simulink model "Simulation_Fahrmodell_v3"  (R2023b)
settings: Solver=ode14x  StartTime=0.0  StopTime=600  FixedStep=0.005  RelTol=1e-3
values from neighbouring files (symbols this model uses):
  bat = bat.computePack()    [DoE_main.m]    (also in DoE_main_sensitivity.m)
  cp = cp.computeP4Map(val_P4, 0, val_P4_DM, 0, 0)    [DoE_main.m]    (also in DoE_main_sensitivity.m = cp.computeP4Map(P4, E2, P4_DM, E3, E4))
  gb = gb.computeShiftMaps()    [DoE_main.m]    (also in DoE_main_sensitivity.m)
  P4 = cfgNum(cfg, 'P4', 0)    [DoE_main_sensitivity.m]    (also in PowertrainConfig.m = 0)
  P4_DM = cfgNum(cfg, 'P4_DM', 0)    [DoE_main_sensitivity.m]    (also in PowertrainConfig.m = 0)
  pt = pt.setupHybrid()    [DoE_main.m]    (also in DoE_main_sensitivity.m)
  veh = VehicleConfig()    [DoE_main.m]    (also in DoE_main_sensitivity.m)
undefined symbols (not defined in the file or in its folder): cp_Zelle_JpkgK, Ice_derfacLoadDecrease_MAP, Ice_derfacLoadIncrease_MAP, Ice_n_axis, Ice_relLoadMax_CUR_n, Ice_relLoadMax_CUR_val, Ice_rl_axis_norm, seconds, SKO_STREET_CHAL, SKO_WHEEL_TYP_CHAL, slip_pacejka, T_init_degC, Track, TT_sliced, use_turbo_model, v_Fzg_init_kmph
libraries: nesl_utility x15, fl_lib x9
(part 5 of 6)

== system Simulation_Fahrmodell_v3/Vehicle Dynamics Model /Drivetrain/Primary and Secondary Axle Powertrain Selector/Primary Axle Powertrain Selector/Hybrid Drive/P2/P2 Motor/Battery and Operating Strategy Limitation (Drive) ==
  Motordrehzahl (1/min) : Inport
  tq_sh_P2_limted : Inport  Port=2
  P_max_EM_kW : Inport  Port=3
  "Begrenzung BAT + Betriebsstrategie EM P2, Fahren1" : Subsystem
  Discharge Limit : Subsystem
  n_Upmin OUT : Outport
  tq_sh_P2_bat_limted : Outport  Port=2
  wires:
  "Begrenzung BAT + Betriebsstrategie EM P2, Fahren1"/2(M_begr_Nm) -> tq_sh_P2_bat_limted/1  "P2_M_Nm_Fahren"
  tq_sh_P2_limted/1 -> Discharge Limit/1(Torque_Drive_In)
  Motordrehzahl (1/min)/1 -> "Begrenzung BAT + Betriebsstrategie EM P2, Fahren1"/1(n_Upmin IN)
  Discharge Limit/1(Torque_Drive_Out) -> "Begrenzung BAT + Betriebsstrategie EM P2, Fahren1"/2(M_Nm)  "P2_M_Nm_Fahren"
  P_max_EM_kW/1 -> "Begrenzung BAT + Betriebsstrategie EM P2, Fahren1"/3(P_mech_max_kW)
  "Begrenzung BAT + Betriebsstrategie EM P2, Fahren1"/1(n_Upmin OUT) -> n_Upmin OUT/1

== system Simulation_Fahrmodell_v3/Vehicle Dynamics Model /Drivetrain/Primary and Secondary Axle Powertrain Selector/Primary Axle Powertrain Selector/Hybrid Drive/P2/P2 Motor/Battery and Operating Strategy Limitation (Recuperation) ==
  Motordrehzahl (1/min) : Inport
  Torque_Recu_In : Inport  Port=2
  P_min_EM_kW : Inport  Port=3
  "Begrenzung BAT + Betriebsstrategie EM P2, Reku1" : Subsystem
  Recuperation Limit1 : Subsystem
  n_Upmin OUT : Outport
  tq_sh_P2_bat_limted_recu : Outport  Port=2
  wires:
  Recuperation Limit1/1(Torque_Recu_Out) -> "Begrenzung BAT + Betriebsstrategie EM P2, Reku1"/2(M_Nm)  "P2_M_Nm_Reku"
  Torque_Recu_In/1 -> Recuperation Limit1/1(Torque_Recu_In)
  "Begrenzung BAT + Betriebsstrategie EM P2, Reku1"/2(M_begr_Nm) -> tq_sh_P2_bat_limted_recu/1  "P2_M_Nm_Reku"
  P_min_EM_kW/1 -> "Begrenzung BAT + Betriebsstrategie EM P2, Reku1"/3(P_mech_max_kW)
  Motordrehzahl (1/min)/1 -> "Begrenzung BAT + Betriebsstrategie EM P2, Reku1"/1(n_Upmin IN)
  "Begrenzung BAT + Betriebsstrategie EM P2, Reku1"/1(n_Upmin OUT) -> n_Upmin OUT/1

== system Simulation_Fahrmodell_v3/Vehicle Dynamics Model /Drivetrain/Primary and Secondary Axle Powertrain Selector/Primary Axle Powertrain Selector/Hybrid Drive/P2/P2 Motor/Power Calculation ==
  n_Upmin : Inport
  tq_sh_P2_bat_limted : Inport  Port=2
  Constant1 : Constant  Value=2*pi/60/1000
  Product : Product  Inputs=3
  P_kW : Outport
  wires:
  Product/1 -> P_kW/1
  n_Upmin/1 -> Product/2
  Constant1/1 -> Product/3
  tq_sh_P2_bat_limted/1 -> Product/1

== system Simulation_Fahrmodell_v3/Vehicle Dynamics Model /Drivetrain/Primary and Secondary Axle Powertrain Selector/Primary Axle Powertrain Selector/Hybrid Drive/P2/P2 Motor/Power Calculation  ==
  n_Upmin : Inport
  tq_sh_P2_bat_limted_recu : Inport  Port=2
  Constant1 : Constant  Value=2*pi/60/1000
  Product : Product  Inputs=3
  P_kW : Outport
  wires:
  Product/1 -> P_kW/1
  n_Upmin/1 -> Product/2
  Constant1/1 -> Product/3
  tq_sh_P2_bat_limted_recu/1 -> Product/1

== system Simulation_Fahrmodell_v3/Vehicle Dynamics Model /Drivetrain/Primary and Secondary Axle Powertrain Selector/Primary Axle Powertrain Selector/Hybrid Drive/P3/P3 Motor/Battery and Operating Strategy Limitation (Drive) ==
  n_Upmin IN : Inport
  tq_sh_P3_limted : Inport  Port=2
  P_max_EM_kW : Inport  Port=3
  "Begrenzung BAT + Betriebsstrategie EM P2, Fahren1" : Subsystem
  Discharge Limit : Subsystem
  n_Upmin OUT : Outport
  tq_sh_P3_bat_limted : Outport  Port=2
  wires:
  P_max_EM_kW/1 -> "Begrenzung BAT + Betriebsstrategie EM P2, Fahren1"/3(P_max_EM_kW)
  tq_sh_P3_limted/1 -> Discharge Limit/1(Torque_Drive_In)
  Discharge Limit/1(Torque_Drive_Out) -> "Begrenzung BAT + Betriebsstrategie EM P2, Fahren1"/2(M_Nm)  "P4_M_Nm_Fahren"
  n_Upmin IN/1 -> "Begrenzung BAT + Betriebsstrategie EM P2, Fahren1"/1(n_Upmin IN)
  "Begrenzung BAT + Betriebsstrategie EM P2, Fahren1"/2(tq_sh_P3_bat_limted) -> tq_sh_P3_bat_limted/1
  "Begrenzung BAT + Betriebsstrategie EM P2, Fahren1"/1(n_Upmin OUT) -> n_Upmin OUT/1

== system Simulation_Fahrmodell_v3/Vehicle Dynamics Model /Drivetrain/Primary and Secondary Axle Powertrain Selector/Primary Axle Powertrain Selector/Hybrid Drive/P3/P3 Motor/Battery and Operating Strategy Limitation (Recuperation) ==
  n_Upmin IN : Inport
  Torque_Recu_In : Inport  Port=2
  P_mech_max_kW : Inport  Port=3
  "Begrenzung BAT + Betriebsstrategie EM P2, Reku1" : Subsystem
  Recuperation Limit1 : Subsystem
  n_Upmin OUT : Outport
  tq_sh_P3_bat_limted : Outport  Port=2
  wires:
  Recuperation Limit1/1(Torque_Recu_Out) -> "Begrenzung BAT + Betriebsstrategie EM P2, Reku1"/2(M_Nm)  "P3_M_Nm_Reu"
  Torque_Recu_In/1 -> Recuperation Limit1/1(Torque_Recu_In)
  n_Upmin IN/1 -> "Begrenzung BAT + Betriebsstrategie EM P2, Reku1"/1(n_Upmin IN)
  "Begrenzung BAT + Betriebsstrategie EM P2, Reku1"/2(M_begr_Nm) -> tq_sh_P3_bat_limted/1
  P_mech_max_kW/1 -> "Begrenzung BAT + Betriebsstrategie EM P2, Reku1"/3(P_mech_max_kW)
  "Begrenzung BAT + Betriebsstrategie EM P2, Reku1"/1(n_Upmin OUT) -> n_Upmin OUT/1

== system Simulation_Fahrmodell_v3/Vehicle Dynamics Model /Drivetrain/Primary and Secondary Axle Powertrain Selector/Primary Axle Powertrain Selector/Hybrid Drive/P3/P3 Motor/Power Calculation ==
  n_Upmin : Inport
  tq_sh_P3_bat_limted : Inport  Port=2
  Constant1 : Constant  Value=2*pi/60/1000
  Product : Product  Inputs=3
  P_max_EM_P3_kW : Outport
  wires:
  Product/1 -> P_max_EM_P3_kW/1
  n_Upmin/1 -> Product/2
  Constant1/1 -> Product/3
  tq_sh_P3_bat_limted/1 -> Product/1

== system Simulation_Fahrmodell_v3/Vehicle Dynamics Model /Drivetrain/Primary and Secondary Axle Powertrain Selector/Primary Axle Powertrain Selector/Hybrid Drive/P3/P3 Motor/Power Calculation  ==
  n_Upmin : Inport
  tq_sh_P3_bat_limted : Inport  Port=2
  Constant1 : Constant  Value=2*pi/60/1000
  Product : Product  Inputs=3
  P_kW : Outport
  wires:
  Product/1 -> P_kW/1
  n_Upmin/1 -> Product/2
  Constant1/1 -> Product/3
  tq_sh_P3_bat_limted/1 -> Product/1

== system Simulation_Fahrmodell_v3/Vehicle Dynamics Model /Drivetrain/Primary and Secondary Axle Powertrain Selector/Secondary Axle Powertrain Selector/Auswahl P4, P4_Dual-Motor/P4 // E2 Single Motor/Battery and Operating Strategy Limitation (Drive)/Begrenzung BAT + Betriebsstrategie EM P4, Fahren1 ==
  n_Upmin IN : Inport
  M_Nm : Inport  Port=2
  P_mech_max_kW : Inport  Port=3
  Max1 : MinMax  Inputs=2
  "P_kW -> M_Nm" : Subsystem
  n_Upmin OUT : Outport
  M_begr_Nm : Outport  Port=2
  wires:
  M_Nm/1 -> Max1/1
  Max1/1 -> M_begr_Nm/1
  "P_kW -> M_Nm"/1(Out1) -> Max1/2  "M_mech_max_Nm"
  n_Upmin IN/1 -> "P_kW -> M_Nm"/2(In2), n_Upmin OUT/1
  P_mech_max_kW/1 -> "P_kW -> M_Nm"/1(P_kW)  "P_kW"

== system Simulation_Fahrmodell_v3/Vehicle Dynamics Model /Drivetrain/Primary and Secondary Axle Powertrain Selector/Secondary Axle Powertrain Selector/Auswahl P4, P4_Dual-Motor/P4 // E2 Single Motor/Battery and Operating Strategy Limitation (Drive)/Discharge Limit ==
  Torque_Drive_In : Inport
  Gain2 : Gain  Gain=100
  MATLAB Function : MATLAB Function  TreatAsAtomicUnit=on
  Recuperation Limit2 : Constant  Value=bat.SOC_Bat_Discharge_Limit
  Torque_Drive_Out : Outport
  wires:
  Torque_Drive_In/1 -> MATLAB Function/1(Torque_In)
  Recuperation Limit2/1 -> Gain2/1
  MATLAB Function/1(Torque_Out) -> Torque_Drive_Out/1
  [SOC] -> MATLAB Function/2(SOC)
  Gain2/1 -> MATLAB Function/3(Discharge_Limit)

== system Simulation_Fahrmodell_v3/Vehicle Dynamics Model /Drivetrain/Primary and Secondary Axle Powertrain Selector/Secondary Axle Powertrain Selector/Auswahl P4, P4_Dual-Motor/P4 // E2 Single Motor/Battery and Operating Strategy Limitation (Recuperation)/Begrenzung BAT + Betriebsstrategie EM P4, Reku1 ==
  n_Upmin IN : Inport
  M_Nm : Inport  Port=2
  P_mech_max_kW : Inport  Port=3
  Max1 : MinMax  Function=max  Inputs=2
  "P_kW -> M_Nm" : Subsystem
  n_Upmin OUT : Outport
  M_begr_Nm : Outport  Port=2
  wires:
  M_Nm/1 -> Max1/1
  Max1/1 -> M_begr_Nm/1
  "P_kW -> M_Nm"/1(Out1) -> Max1/2  "M_mech_max_Nm"
  n_Upmin IN/1 -> "P_kW -> M_Nm"/2(In2), n_Upmin OUT/1
  P_mech_max_kW/1 -> "P_kW -> M_Nm"/1(P_kW)  "P_kW"

== system Simulation_Fahrmodell_v3/Vehicle Dynamics Model /Drivetrain/Primary and Secondary Axle Powertrain Selector/Secondary Axle Powertrain Selector/Auswahl P4, P4_Dual-Motor/P4 // E2 Single Motor/Battery and Operating Strategy Limitation (Recuperation)/Recuperation Limit ==
  Torque_Recu_In : Inport
  Constant : Constant  Value=0
  Gain5 : Gain  Gain=100
  Recuperation Limit : Constant  Value=bat.SOC_Recup_Limit
  Relational Operator2 : RelationalOperator  Operator=<  OutDataTypeStr=boolean  RndMeth=Simplest  InputSameDT=off
  Switch2 : Switch  Criteria=u2 > Threshold  SaturateOnIntegerOverflow=off  InputSameDT=off
  Torque_Recu_Out : Outport
  wires:
  Constant/1 -> Switch2/3
  [SOC] -> Relational Operator2/1
  Recuperation Limit/1 -> Gain5/1
  Relational Operator2/1 -> Switch2/2
  Torque_Recu_In/1 -> Switch2/1
  Switch2/1 -> Torque_Recu_Out/1
  Gain5/1 -> Relational Operator2/2

== system Simulation_Fahrmodell_v3/Vehicle Dynamics Model /Drivetrain/Primary and Secondary Axle Powertrain Selector/Secondary Axle Powertrain Selector/Auswahl P4, P4_Dual-Motor/P4 // E3 // E4 Dual Motor/Battery and Operating Strategy Limitation (Drive) 1/Begrenzung BAT + Betriebsstrategie EM P4_DM_L, Fahren1 ==
  n_Upmin IN : Inport
  M_Nm : Inport  Port=2
  P_mech_max_kW : Inport  Port=3
  Max1 : MinMax  Inputs=2
  "P_kW -> M_Nm" : Subsystem
  n_Upmin OUT : Outport
  M_begr_Nm : Outport  Port=2
  wires:
  M_Nm/1 -> Max1/1
  Max1/1 -> M_begr_Nm/1
  "P_kW -> M_Nm"/1(Out1) -> Max1/2  "M_mech_max_Nm"
  n_Upmin IN/1 -> "P_kW -> M_Nm"/2(In2), n_Upmin OUT/1
  P_mech_max_kW/1 -> "P_kW -> M_Nm"/1(P_kW)  "P_kW"

== system Simulation_Fahrmodell_v3/Vehicle Dynamics Model /Drivetrain/Primary and Secondary Axle Powertrain Selector/Secondary Axle Powertrain Selector/Auswahl P4, P4_Dual-Motor/P4 // E3 // E4 Dual Motor/Battery and Operating Strategy Limitation (Drive) 1/Discharge Limit1 ==
  Torque_Drive_In : Inport
  Gain2 : Gain  Gain=100
  MATLAB Function : MATLAB Function  TreatAsAtomicUnit=on
  Recuperation Limit2 : Constant  Value=bat.SOC_Bat_Discharge_Limit
  Torque_Drive_Out : Outport
  wires:
  Torque_Drive_In/1 -> MATLAB Function/1(Torque_In)
  Recuperation Limit2/1 -> Gain2/1
  MATLAB Function/1(Torque_Out) -> Torque_Drive_Out/1
  [SOC] -> MATLAB Function/2(SOC)
  Gain2/1 -> MATLAB Function/3(Discharge_Limit)

== system Simulation_Fahrmodell_v3/Vehicle Dynamics Model /Drivetrain/Primary and Secondary Axle Powertrain Selector/Secondary Axle Powertrain Selector/Auswahl P4, P4_Dual-Motor/P4 // E3 // E4 Dual Motor/Battery and Operating Strategy Limitation (Drive) 2/Begrenzung BAT + Betriebsstrategie EM P4_DM_R, Fahren2 ==
  n_Upmin IN : Inport
  M_Nm : Inport  Port=2
  P_mech_max_kW : Inport  Port=3
  Max1 : MinMax  Inputs=2
  "P_kW -> M_Nm" : Subsystem
  n_Upmin OUT : Outport
  M_begr_Nm : Outport  Port=2
  wires:
  M_Nm/1 -> Max1/1
  Max1/1 -> M_begr_Nm/1
  "P_kW -> M_Nm"/1(Out1) -> Max1/2  "M_mech_max_Nm"
  n_Upmin IN/1 -> "P_kW -> M_Nm"/2(In2), n_Upmin OUT/1
  P_mech_max_kW/1 -> "P_kW -> M_Nm"/1(P_kW)  "P_kW"

== system Simulation_Fahrmodell_v3/Vehicle Dynamics Model /Drivetrain/Primary and Secondary Axle Powertrain Selector/Secondary Axle Powertrain Selector/Auswahl P4, P4_Dual-Motor/P4 // E3 // E4 Dual Motor/Battery and Operating Strategy Limitation (Drive) 2/Discharge Limit ==
  Torque_Drive_In : Inport
  Gain2 : Gain  Gain=100
  MATLAB Function : MATLAB Function  TreatAsAtomicUnit=on
  Recuperation Limit2 : Constant  Value=bat.SOC_Bat_Discharge_Limit
  Torque_Drive_Out : Outport
  wires:
  Torque_Drive_In/1 -> MATLAB Function/1(Torque_In)
  Recuperation Limit2/1 -> Gain2/1
  MATLAB Function/1(Torque_Out) -> Torque_Drive_Out/1
  [SOC] -> MATLAB Function/2(SOC)
  Gain2/1 -> MATLAB Function/3(Discharge_Limit)

== system Simulation_Fahrmodell_v3/Vehicle Dynamics Model /Drivetrain/Primary and Secondary Axle Powertrain Selector/Secondary Axle Powertrain Selector/Auswahl P4, P4_Dual-Motor/P4 // E3 // E4 Dual Motor/Battery and Operating Strategy Limitation (Recuperation) 1/Begrenzung BAT + Betriebsstrategie EM P4_DM_L, Reku1 ==
  n_Upmin IN : Inport
  M_Nm : Inport  Port=2
  P_mech_max_kW : Inport  Port=3
  Max1 : MinMax  Function=max  Inputs=2
  "P_kW -> M_Nm" : Subsystem
  n_Upmin OUT : Outport
  M_begr_Nm : Outport  Port=2
  wires:
  M_Nm/1 -> Max1/1
  Max1/1 -> M_begr_Nm/1
  "P_kW -> M_Nm"/1(Out1) -> Max1/2  "M_mech_max_Nm"
  n_Upmin IN/1 -> "P_kW -> M_Nm"/2(In2), n_Upmin OUT/1
  P_mech_max_kW/1 -> "P_kW -> M_Nm"/1(P_kW)  "P_kW"

== system Simulation_Fahrmodell_v3/Vehicle Dynamics Model /Drivetrain/Primary and Secondary Axle Powertrain Selector/Secondary Axle Powertrain Selector/Auswahl P4, P4_Dual-Motor/P4 // E3 // E4 Dual Motor/Battery and Operating Strategy Limitation (Recuperation) 1/Recuperation Limit1 ==
  Torque_Recu_In : Inport
  Constant : Constant  Value=0
  Gain5 : Gain  Gain=100
  Recuperation Limit : Constant  Value=bat.SOC_Recup_Limit
  Relational Operator2 : RelationalOperator  Operator=<  OutDataTypeStr=boolean  RndMeth=Simplest  InputSameDT=off
  Switch2 : Switch  Criteria=u2 > Threshold  SaturateOnIntegerOverflow=off  InputSameDT=off
  Torque_Recu_Out : Outport
  wires:
  Constant/1 -> Switch2/3
  [SOC] -> Relational Operator2/1
  Recuperation Limit/1 -> Gain5/1
  Relational Operator2/1 -> Switch2/2
  Torque_Recu_In/1 -> Switch2/1
  Switch2/1 -> Torque_Recu_Out/1
  Gain5/1 -> Relational Operator2/2

== system Simulation_Fahrmodell_v3/Vehicle Dynamics Model /Drivetrain/Primary and Secondary Axle Powertrain Selector/Secondary Axle Powertrain Selector/Auswahl P4, P4_Dual-Motor/P4 // E3 // E4 Dual Motor/Battery and Operating Strategy Limitation (Recuperation) 2/Begrenzung BAT + Betriebsstrategie EM P4_DM_R, Reku2 ==
  n_Upmin IN : Inport
  M_Nm : Inport  Port=2
  P_mech_max_kW : Inport  Port=3
  Max1 : MinMax  Function=max  Inputs=2
  "P_kW -> M_Nm" : Subsystem
  n_Upmin OUT : Outport
  M_begr_Nm : Outport  Port=2
  wires:
  M_Nm/1 -> Max1/1
  Max1/1 -> M_begr_Nm/1
  "P_kW -> M_Nm"/1(Out1) -> Max1/2  "M_mech_max_Nm"
  n_Upmin IN/1 -> "P_kW -> M_Nm"/2(In2), n_Upmin OUT/1
  P_mech_max_kW/1 -> "P_kW -> M_Nm"/1(P_kW)  "P_kW"

== system Simulation_Fahrmodell_v3/Vehicle Dynamics Model /Drivetrain/Primary and Secondary Axle Powertrain Selector/Secondary Axle Powertrain Selector/Auswahl P4, P4_Dual-Motor/P4 // E3 // E4 Dual Motor/Battery and Operating Strategy Limitation (Recuperation) 2/Recuperation Limit ==
  Torque_Recu_In : Inport
  Constant : Constant  Value=0
  Gain5 : Gain  Gain=100
  Recuperation Limit : Constant  Value=bat.SOC_Recup_Limit
  Relational Operator2 : RelationalOperator  Operator=<  OutDataTypeStr=boolean  RndMeth=Simplest  InputSameDT=off
  Switch2 : Switch  Criteria=u2 > Threshold  SaturateOnIntegerOverflow=off  InputSameDT=off
  Torque_Recu_Out : Outport
  wires:
  Constant/1 -> Switch2/3
  [SOC] -> Relational Operator2/1
  Recuperation Limit/1 -> Gain5/1
  Relational Operator2/1 -> Switch2/2
  Torque_Recu_In/1 -> Switch2/1
  Switch2/1 -> Torque_Recu_Out/1
  Gain5/1 -> Relational Operator2/2

== system Simulation_Fahrmodell_v3/Vehicle Dynamics Model /Drivetrain/Primary and Secondary Axle Powertrain Selector/Primary Axle Powertrain Selector/Electric Drive/Variant Subsystem/EV Dual Motor/Battery and Operating Strategy Limitation (Drive)/Begrenzung BAT + Betriebsstrategie EM P4_DM_L, Fahren2 ==
  n_Upmin IN : Inport
  M_Nm : Inport  Port=2
  P_mech_max_kW : Inport  Port=3
  Max1 : MinMax  Inputs=2
  "P_kW -> M_Nm" : Subsystem
  n_Upmin OUT : Outport
  M_begr_Nm : Outport  Port=2
  wires:
  M_Nm/1 -> Max1/1
  Max1/1 -> M_begr_Nm/1
  "P_kW -> M_Nm"/1(Out1) -> Max1/2  "M_mech_max_Nm"
  n_Upmin IN/1 -> "P_kW -> M_Nm"/2(In2), n_Upmin OUT/1
  P_mech_max_kW/1 -> "P_kW -> M_Nm"/1(P_kW)  "P_kW"

== system Simulation_Fahrmodell_v3/Vehicle Dynamics Model /Drivetrain/Primary and Secondary Axle Powertrain Selector/Primary Axle Powertrain Selector/Electric Drive/Variant Subsystem/EV Dual Motor/Battery and Operating Strategy Limitation (Drive)/Discharge Limit ==
  Torque_Drive_In : Inport
  Gain2 : Gain  Gain=100
  MATLAB Function : MATLAB Function  TreatAsAtomicUnit=on
  Recuperation Limit2 : Constant  Value=bat.SOC_Bat_Discharge_Limit
  Torque_Drive_Out : Outport
  wires:
  Torque_Drive_In/1 -> MATLAB Function/1(Torque_In)
  MATLAB Function/1(Torque_Out) -> Torque_Drive_Out/1
  [SOC] -> MATLAB Function/2(SOC)
  Recuperation Limit2/1 -> Gain2/1
  Gain2/1 -> MATLAB Function/3(Discharge_Limit)

== system Simulation_Fahrmodell_v3/Vehicle Dynamics Model /Drivetrain/Primary and Secondary Axle Powertrain Selector/Primary Axle Powertrain Selector/Electric Drive/Variant Subsystem/EV Dual Motor/Battery and Operating Strategy Limitation (Drive) /Begrenzung BAT + Betriebsstrategie EM P4_DM_R, Fahren1 ==
  n_Upmin IN : Inport
  M_Nm : Inport  Port=2
  P_mech_max_kW : Inport  Port=3
  Max1 : MinMax  Inputs=2
  "P_kW -> M_Nm" : Subsystem
  n_Upmin OUT : Outport
  M_begr_Nm : Outport  Port=2
  wires:
  M_Nm/1 -> Max1/1
  Max1/1 -> M_begr_Nm/1
  "P_kW -> M_Nm"/1(Out1) -> Max1/2  "M_mech_max_Nm"
  n_Upmin IN/1 -> "P_kW -> M_Nm"/2(In2), n_Upmin OUT/1
  P_mech_max_kW/1 -> "P_kW -> M_Nm"/1(P_kW)  "P_kW"

== system Simulation_Fahrmodell_v3/Vehicle Dynamics Model /Drivetrain/Primary and Secondary Axle Powertrain Selector/Primary Axle Powertrain Selector/Electric Drive/Variant Subsystem/EV Dual Motor/Battery and Operating Strategy Limitation (Drive) /Discharge Limit1 ==
  Torque_Drive_In : Inport
  Add : Sum  Commented=on
  Constant : Constant  Commented=on  Value=0
  Constant1 : Constant  Commented=on  Value=10
  From1 : From  Commented=on  GotoTag=SOC  TagVisibility=global
  From8 : From  Commented=on  GotoTag=SOC  TagVisibility=global
  Gain1 : Gain  Commented=on  Gain=100
  Gain2 : Gain  Gain=100
  Gain5 : Gain  Commented=on  Gain=100
  MATLAB Function : MATLAB Function  TreatAsAtomicUnit=on
  Recuperation Limit : Constant  Commented=on  Value=bat.SOC_Bat_Discharge_Limit
  Recuperation Limit1 : Constant  Commented=on  Value=bat.SOC_Bat_Discharge_Limit
  Recuperation Limit2 : Constant  Value=bat.SOC_Bat_Discharge_Limit
  Relational Operator1 : RelationalOperator  Commented=on  Operator=>  OutDataTypeStr=boolean  RndMeth=Simplest  InputSameDT=off
  Relational Operator2 : RelationalOperator  Commented=on  Operator=>  OutDataTypeStr=boolean  RndMeth=Simplest  InputSameDT=off
  Switch1 : Switch  Commented=on  Criteria=u2 > Threshold  SaturateOnIntegerOverflow=off  InputSameDT=off
  Switch2 : Switch  Commented=on  Criteria=u2 > Threshold  SaturateOnIntegerOverflow=off  InputSameDT=off
  Torque_Drive_Out : Outport
  wires:
  Switch1/1 -> ?
  Recuperation Limit1/1 -> Gain1/1
  Add/1 -> Relational Operator1/2
  Relational Operator1/1 -> Switch1/2
  From1/1 -> Relational Operator1/1
  Gain1/1 -> Add/1
  Switch2/1 -> Switch1/1
  ? -> Switch2/1
  Recuperation Limit/1 -> Gain5/1
  Constant/1 -> Switch2/3, Switch1/3
  From8/1 -> Relational Operator2/1
  Relational Operator2/1 -> Switch2/2
  Constant1/1 -> Add/2
  Gain5/1 -> Relational Operator2/2
  Torque_Drive_In/1 -> MATLAB Function/1(Torque_In)
  Recuperation Limit2/1 -> Gain2/1
  MATLAB Function/1(Torque_Out) -> Torque_Drive_Out/1
  [SOC] -> MATLAB Function/2(SOC)
  Gain2/1 -> MATLAB Function/3(Discharge_Limit)

== system Simulation_Fahrmodell_v3/Vehicle Dynamics Model /Drivetrain/Primary and Secondary Axle Powertrain Selector/Primary Axle Powertrain Selector/Electric Drive/Variant Subsystem/EV Dual Motor/Battery and Operating Strategy Limitation (Recuperation)/Begrenzung BAT + Betriebsstrategie EM P4_DM_L, Reku2 ==
  n_Upmin IN : Inport
  M_Nm : Inport  Port=2
  P_mech_max_kW : Inport  Port=3
  Max1 : MinMax  Function=max  Inputs=2
  "P_kW -> M_Nm" : Subsystem
  n_Upmin OUT : Outport
  M_begr_Nm : Outport  Port=2
  wires:
  M_Nm/1 -> Max1/1
  Max1/1 -> M_begr_Nm/1
  "P_kW -> M_Nm"/1(Out1) -> Max1/2  "M_mech_max_Nm"
  n_Upmin IN/1 -> "P_kW -> M_Nm"/2(In2), n_Upmin OUT/1
  P_mech_max_kW/1 -> "P_kW -> M_Nm"/1(P_kW)  "P_kW"

== system Simulation_Fahrmodell_v3/Vehicle Dynamics Model /Drivetrain/Primary and Secondary Axle Powertrain Selector/Primary Axle Powertrain Selector/Electric Drive/Variant Subsystem/EV Dual Motor/Battery and Operating Strategy Limitation (Recuperation)/Recuperation Limit1 ==
  Torque_Recu_In : Inport
  Constant : Constant  Value=0
  Gain5 : Gain  Gain=100
  Recuperation Limit : Constant  Value=bat.SOC_Recup_Limit
  Relational Operator2 : RelationalOperator  Operator=<  OutDataTypeStr=boolean  RndMeth=Simplest  InputSameDT=off
  Switch2 : Switch  Criteria=u2 > Threshold  SaturateOnIntegerOverflow=off  InputSameDT=off
  Torque_Recu_Out : Outport
  wires:
  Constant/1 -> Switch2/3
  [SOC] -> Relational Operator2/1
  Recuperation Limit/1 -> Gain5/1
  Relational Operator2/1 -> Switch2/2
  Torque_Recu_In/1 -> Switch2/1
  Switch2/1 -> Torque_Recu_Out/1
  Gain5/1 -> Relational Operator2/2

== system Simulation_Fahrmodell_v3/Vehicle Dynamics Model /Drivetrain/Primary and Secondary Axle Powertrain Selector/Primary Axle Powertrain Selector/Electric Drive/Variant Subsystem/EV Dual Motor/Battery and Operating Strategy Limitation (Recuperation) /Begrenzung BAT + Betriebsstrategie EM P4_DM_R, Reku1 ==
  n_Upmin IN : Inport
  M_Nm : Inport  Port=2
  P_mech_max_kW : Inport  Port=3
  Max1 : MinMax  Function=max  Inputs=2
  "P_kW -> M_Nm" : Subsystem
  n_Upmin OUT : Outport
  M_begr_Nm : Outport  Port=2
  wires:
  M_Nm/1 -> Max1/1
  Max1/1 -> M_begr_Nm/1
  "P_kW -> M_Nm"/1(Out1) -> Max1/2  "M_mech_max_Nm"
  n_Upmin IN/1 -> "P_kW -> M_Nm"/2(In2), n_Upmin OUT/1
  P_mech_max_kW/1 -> "P_kW -> M_Nm"/1(P_kW)  "P_kW"

== system Simulation_Fahrmodell_v3/Vehicle Dynamics Model /Drivetrain/Primary and Secondary Axle Powertrain Selector/Primary Axle Powertrain Selector/Electric Drive/Variant Subsystem/EV Dual Motor/Battery and Operating Strategy Limitation (Recuperation) /Recuperation Limit ==
  Torque_Recu_In : Inport
  Constant : Constant  Value=0
  Gain5 : Gain  Gain=100
  Recuperation Limit : Constant  Value=bat.SOC_Recup_Limit
  Relational Operator2 : RelationalOperator  Operator=<  OutDataTypeStr=boolean  RndMeth=Simplest  InputSameDT=off
  Switch2 : Switch  Criteria=u2 > Threshold  SaturateOnIntegerOverflow=off  InputSameDT=off
  Torque_Recu_Out : Outport
  wires:
  Constant/1 -> Switch2/3
  [SOC] -> Relational Operator2/1
  Recuperation Limit/1 -> Gain5/1
  Relational Operator2/1 -> Switch2/2
  Torque_Recu_In/1 -> Switch2/1
  Switch2/1 -> Torque_Recu_Out/1
  Gain5/1 -> Relational Operator2/2

== system Simulation_Fahrmodell_v3/Vehicle Dynamics Model /Drivetrain/Primary and Secondary Axle Powertrain Selector/Primary Axle Powertrain Selector/Electric Drive/Variant Subsystem/EV Single Motor/Battery and Operating Strategy Limitation (Drive)/Begrenzung BAT + Betriebsstrategie EM EV, Fahren2 ==
  n_Upmin IN : Inport
  M_Nm : Inport  Port=2
  P_mech_max_kW : Inport  Port=3
  Max1 : MinMax  Inputs=2
  "P_kW -> M_Nm" : Subsystem
  n_Upmin OUT : Outport
  M_begr_Nm : Outport  Port=2
  wires:
  M_Nm/1 -> Max1/1
  Max1/1 -> M_begr_Nm/1
  "P_kW -> M_Nm"/1(Out1) -> Max1/2  "M_mech_max_Nm"
  n_Upmin IN/1 -> "P_kW -> M_Nm"/2(In2), n_Upmin OUT/1
  P_mech_max_kW/1 -> "P_kW -> M_Nm"/1(P_kW)  "P_kW"

== system Simulation_Fahrmodell_v3/Vehicle Dynamics Model /Drivetrain/Primary and Secondary Axle Powertrain Selector/Primary Axle Powertrain Selector/Electric Drive/Variant Subsystem/EV Single Motor/Battery and Operating Strategy Limitation (Drive)/Discharge Limit ==
  Torque_Drive_In : Inport
  Gain2 : Gain  Gain=100
  MATLAB Function : MATLAB Function  TreatAsAtomicUnit=on
  Recuperation Limit2 : Constant  Value=bat.SOC_Bat_Discharge_Limit
  Torque_Drive_Out : Outport
  wires:
  Torque_Drive_In/1 -> MATLAB Function/1(Torque_In)
  Recuperation Limit2/1 -> Gain2/1
  MATLAB Function/1(Torque_Out) -> Torque_Drive_Out/1
  [SOC] -> MATLAB Function/2(SOC)
  Gain2/1 -> MATLAB Function/3(Discharge_Limit)

== system Simulation_Fahrmodell_v3/Vehicle Dynamics Model /Drivetrain/Primary and Secondary Axle Powertrain Selector/Primary Axle Powertrain Selector/Electric Drive/Variant Subsystem/EV Single Motor/Battery and Operating Strategy Limitation (Recuperation)/Begrenzung BAT + Betriebsstrategie EM EV, Reku2 ==
  n_Upmin IN : Inport
  M_Nm : Inport  Port=2
  P_mech_max_kW : Inport  Port=3
  Max1 : MinMax  Function=max  Inputs=2
  "P_kW -> M_Nm" : Subsystem
  n_Upmin OUT : Outport
  M_begr_Nm : Outport  Port=2
  wires:
  M_Nm/1 -> Max1/1
  Max1/1 -> M_begr_Nm/1
  "P_kW -> M_Nm"/1(Out1) -> Max1/2  "M_mech_max_Nm"
  n_Upmin IN/1 -> "P_kW -> M_Nm"/2(In2), n_Upmin OUT/1
  P_mech_max_kW/1 -> "P_kW -> M_Nm"/1(P_kW)  "P_kW"

== system Simulation_Fahrmodell_v3/Vehicle Dynamics Model /Drivetrain/Primary and Secondary Axle Powertrain Selector/Primary Axle Powertrain Selector/Electric Drive/Variant Subsystem/EV Single Motor/Battery and Operating Strategy Limitation (Recuperation)/Recuperation Limit ==
  Torque_Recu_In : Inport
  Constant : Constant  Value=0
  Gain5 : Gain  Gain=100
  Recuperation Limit : Constant  Value=bat.SOC_Recup_Limit
  Relational Operator2 : RelationalOperator  Operator=<  OutDataTypeStr=boolean  RndMeth=Simplest  InputSameDT=off
  Switch2 : Switch  Criteria=u2 > Threshold  SaturateOnIntegerOverflow=off  InputSameDT=off
  Torque_Recu_Out : Outport
  wires:
  Constant/1 -> Switch2/3
  [SOC] -> Relational Operator2/1
  Recuperation Limit/1 -> Gain5/1
  Relational Operator2/1 -> Switch2/2
  Torque_Recu_In/1 -> Switch2/1
  Switch2/1 -> Torque_Recu_Out/1
  Gain5/1 -> Relational Operator2/2

== system Simulation_Fahrmodell_v3/Vehicle Dynamics Model /Drivetrain/Primary and Secondary Axle Powertrain Selector/Primary Axle Powertrain Selector/Hybrid Drive/P0/P0 Motor/Battery and Operating Strategy Limitation (Recuperation)/Begrenzung BAT + Betriebsstrategie EM P2, Reku1 ==
  n_Upmin IN : Inport
  M_Nm : Inport  Port=2
  P_mech_max_kW : Inport  Port=3
  Max1 : MinMax  Function=max  Inputs=2
  "P_kW -> M_Nm" : Subsystem
  n_Upmin OUT : Outport
  M_begr_Nm : Outport  Port=2
  wires:
  M_Nm/1 -> Max1/1
  Max1/1 -> M_begr_Nm/1
  "P_kW -> M_Nm"/1(Out1) -> Max1/2  "M_mech_max_Nm"
  n_Upmin IN/1 -> "P_kW -> M_Nm"/2(In2), n_Upmin OUT/1
  P_mech_max_kW/1 -> "P_kW -> M_Nm"/1(P_kW)  "P_kW"

== system Simulation_Fahrmodell_v3/Vehicle Dynamics Model /Drivetrain/Primary and Secondary Axle Powertrain Selector/Primary Axle Powertrain Selector/Hybrid Drive/P0/P0 Motor/Battery and Operating Strategy Limitation (Recuperation)/Recuperation Limit1 ==
  Torque_Recu_In : Inport
  Constant : Constant  Value=0
  Gain5 : Gain  Gain=100
  Recuperation Limit : Constant  Value=bat.SOC_Recup_Limit
  Relational Operator2 : RelationalOperator  Operator=<  OutDataTypeStr=boolean  RndMeth=Simplest  InputSameDT=off
  Switch2 : Switch  Criteria=u2 > Threshold  SaturateOnIntegerOverflow=off  InputSameDT=off
  Torque_Recu_Out : Outport
  wires:
  Constant/1 -> Switch2/3
  [SOC] -> Relational Operator2/1
  Recuperation Limit/1 -> Gain5/1
  Relational Operator2/1 -> Switch2/2
  Torque_Recu_In/1 -> Switch2/1
  Switch2/1 -> Torque_Recu_Out/1
  Gain5/1 -> Relational Operator2/2

== system Simulation_Fahrmodell_v3/Vehicle Dynamics Model /Drivetrain/Primary and Secondary Axle Powertrain Selector/Primary Axle Powertrain Selector/Hybrid Drive/P0/P0 Motor/SubsysteBattery and Operating Strategy Limitation (Drive)m/Begrenzung BAT + Betriebsstrategie EM P2, Fahren1 ==
  n_Upmin IN : Inport
  M_Nm : Inport  Port=2
  P_mech_max_kW : Inport  Port=3
  Max1 : MinMax  Inputs=2
  "P_kW -> M_Nm" : Subsystem
  n_Upmin OUT : Outport
  M_begr_Nm : Outport  Port=2
  wires:
  M_Nm/1 -> Max1/1
  Max1/1 -> M_begr_Nm/1
  "P_kW -> M_Nm"/1(Out1) -> Max1/2  "M_mech_max_Nm"
  n_Upmin IN/1 -> "P_kW -> M_Nm"/2(In2), n_Upmin OUT/1
  P_mech_max_kW/1 -> "P_kW -> M_Nm"/1(P_kW)  "P_kW"

== system Simulation_Fahrmodell_v3/Vehicle Dynamics Model /Drivetrain/Primary and Secondary Axle Powertrain Selector/Primary Axle Powertrain Selector/Hybrid Drive/P0/P0 Motor/SubsysteBattery and Operating Strategy Limitation (Drive)m/Discharge Limit ==
  Torque_Drive_In : Inport
  Gain2 : Gain  Gain=100
  MATLAB Function : MATLAB Function  TreatAsAtomicUnit=on
  Recuperation Limit2 : Constant  Value=bat.SOC_Bat_Discharge_Limit
  Torque_Drive_Out : Outport
  wires:
  Torque_Drive_In/1 -> MATLAB Function/1(Torque_In)
  Recuperation Limit2/1 -> Gain2/1
  MATLAB Function/1(Torque_Out) -> Torque_Drive_Out/1
  [SOC] -> MATLAB Function/2(SOC)
  Gain2/1 -> MATLAB Function/3(Discharge_Limit)

== system Simulation_Fahrmodell_v3/Vehicle Dynamics Model /Drivetrain/Primary and Secondary Axle Powertrain Selector/Primary Axle Powertrain Selector/Hybrid Drive/P2/P2 Motor/Battery and Operating Strategy Limitation (Drive)/Begrenzung BAT + Betriebsstrategie EM P2, Fahren1 ==
  n_Upmin IN : Inport
  M_Nm : Inport  Port=2
  P_mech_max_kW : Inport  Port=3
  Max1 : MinMax  Inputs=2
  "P_kW -> M_Nm" : Subsystem
  n_Upmin OUT : Outport
  M_begr_Nm : Outport  Port=2
  wires:
  M_Nm/1 -> Max1/1
  Max1/1 -> M_begr_Nm/1
  "P_kW -> M_Nm"/1(Out1) -> Max1/2  "M_mech_max_Nm"
  n_Upmin IN/1 -> "P_kW -> M_Nm"/2(In2), n_Upmin OUT/1
  P_mech_max_kW/1 -> "P_kW -> M_Nm"/1(P_kW)  "P_kW"

== system Simulation_Fahrmodell_v3/Vehicle Dynamics Model /Drivetrain/Primary and Secondary Axle Powertrain Selector/Primary Axle Powertrain Selector/Hybrid Drive/P2/P2 Motor/Battery and Operating Strategy Limitation (Drive)/Discharge Limit ==
  Torque_Drive_In : Inport
  Gain2 : Gain  Gain=100
  MATLAB Function : MATLAB Function  TreatAsAtomicUnit=on
  Recuperation Limit2 : Constant  Value=bat.SOC_Bat_Discharge_Limit
  Torque_Drive_Out : Outport
  wires:
  Torque_Drive_In/1 -> MATLAB Function/1(Torque_In)
  Recuperation Limit2/1 -> Gain2/1
  MATLAB Function/1(Torque_Out) -> Torque_Drive_Out/1
  [SOC] -> MATLAB Function/2(SOC)
  Gain2/1 -> MATLAB Function/3(Discharge_Limit)

== system Simulation_Fahrmodell_v3/Vehicle Dynamics Model /Drivetrain/Primary and Secondary Axle Powertrain Selector/Primary Axle Powertrain Selector/Hybrid Drive/P2/P2 Motor/Battery and Operating Strategy Limitation (Recuperation)/Begrenzung BAT + Betriebsstrategie EM P2, Reku1 ==
  n_Upmin IN : Inport
  M_Nm : Inport  Port=2
  P_mech_max_kW : Inport  Port=3
  Max1 : MinMax  Function=max  Inputs=2
  "P_kW -> M_Nm" : Subsystem
  n_Upmin OUT : Outport
  M_begr_Nm : Outport  Port=2
  wires:
  M_Nm/1 -> Max1/1
  Max1/1 -> M_begr_Nm/1
  "P_kW -> M_Nm"/1(Out1) -> Max1/2  "M_mech_max_Nm"
  n_Upmin IN/1 -> "P_kW -> M_Nm"/2(In2), n_Upmin OUT/1
  P_mech_max_kW/1 -> "P_kW -> M_Nm"/1(P_kW)  "P_kW"

== system Simulation_Fahrmodell_v3/Vehicle Dynamics Model /Drivetrain/Primary and Secondary Axle Powertrain Selector/Primary Axle Powertrain Selector/Hybrid Drive/P2/P2 Motor/Battery and Operating Strategy Limitation (Recuperation)/Recuperation Limit1 ==
  Torque_Recu_In : Inport
  Constant : Constant  Value=0
  Gain5 : Gain  Gain=100
  Recuperation Limit : Constant  Value=bat.SOC_Recup_Limit
  Relational Operator2 : RelationalOperator  Operator=<  OutDataTypeStr=boolean  RndMeth=Simplest  InputSameDT=off
  Switch2 : Switch  Criteria=u2 > Threshold  SaturateOnIntegerOverflow=off  InputSameDT=off
  Torque_Recu_Out : Outport
  wires:
  Constant/1 -> Switch2/3
  [SOC] -> Relational Operator2/1
  Recuperation Limit/1 -> Gain5/1
  Relational Operator2/1 -> Switch2/2
  Torque_Recu_In/1 -> Switch2/1
  Switch2/1 -> Torque_Recu_Out/1
  Gain5/1 -> Relational Operator2/2

== system Simulation_Fahrmodell_v3/Vehicle Dynamics Model /Drivetrain/Primary and Secondary Axle Powertrain Selector/Primary Axle Powertrain Selector/Hybrid Drive/P3/P3 Motor/Battery and Operating Strategy Limitation (Drive)/Begrenzung BAT + Betriebsstrategie EM P2, Fahren1 ==
  n_Upmin IN : Inport
  M_Nm : Inport  Port=2
  P_max_EM_kW : Inport  Port=3
  Max1 : MinMax  Inputs=2
  "P_kW -> M_Nm" : Subsystem
  n_Upmin OUT : Outport
  tq_sh_P3_bat_limted : Outport  Port=2
  wires:
  M_Nm/1 -> Max1/1
  Max1/1 -> tq_sh_P3_bat_limted/1
  "P_kW -> M_Nm"/1(Out1) -> Max1/2  "M_max_EM_Nm"
  n_Upmin IN/1 -> "P_kW -> M_Nm"/2(In2), n_Upmin OUT/1
  P_max_EM_kW/1 -> "P_kW -> M_Nm"/1(P_kW)  "P_kW"

== system Simulation_Fahrmodell_v3/Vehicle Dynamics Model /Drivetrain/Primary and Secondary Axle Powertrain Selector/Primary Axle Powertrain Selector/Hybrid Drive/P3/P3 Motor/Battery and Operating Strategy Limitation (Drive)/Discharge Limit ==
  Torque_Drive_In : Inport
  Add : Sum  Commented=on
  Constant : Constant  Commented=on  Value=0
  Constant1 : Constant  Commented=on  Value=10
  From1 : From  Commented=on  GotoTag=SOC  TagVisibility=global
  From8 : From  Commented=on  GotoTag=SOC  TagVisibility=global
  Gain1 : Gain  Commented=on  Gain=100
  Gain2 : Gain  Gain=100
  Gain5 : Gain  Commented=on  Gain=100
  MATLAB Function : MATLAB Function  TreatAsAtomicUnit=on
  Recuperation Limit : Constant  Commented=on  Value=bat.SOC_Bat_Discharge_Limit
  Recuperation Limit1 : Constant  Commented=on  Value=bat.SOC_Bat_Discharge_Limit
  Recuperation Limit2 : Constant  Value=bat.SOC_Bat_Discharge_Limit
  Relational Operator1 : RelationalOperator  Commented=on  Operator=>  OutDataTypeStr=boolean  RndMeth=Simplest  InputSameDT=off
  Relational Operator2 : RelationalOperator  Commented=on  Operator=>  OutDataTypeStr=boolean  RndMeth=Simplest  InputSameDT=off
  Switch1 : Switch  Commented=on  Criteria=u2 > Threshold  SaturateOnIntegerOverflow=off  InputSameDT=off
  Switch2 : Switch  Commented=on  Criteria=u2 > Threshold  SaturateOnIntegerOverflow=off  InputSameDT=off
  Torque_Drive_Out : Outport
  wires:
  Switch1/1 -> ?
  Recuperation Limit1/1 -> Gain1/1
  Add/1 -> Relational Operator1/2
  Relational Operator1/1 -> Switch1/2
  From1/1 -> Relational Operator1/1
  Gain1/1 -> Add/1
  Switch2/1 -> Switch1/1
  ? -> Switch2/1
  Recuperation Limit/1 -> Gain5/1
  Constant/1 -> Switch2/3, Switch1/3
  From8/1 -> Relational Operator2/1
  Relational Operator2/1 -> Switch2/2
  Constant1/1 -> Add/2
  Gain5/1 -> Relational Operator2/2
  Torque_Drive_In/1 -> MATLAB Function/1(Torque_In)
  Recuperation Limit2/1 -> Gain2/1
  MATLAB Function/1(Torque_Out) -> Torque_Drive_Out/1
  [SOC] -> MATLAB Function/2(SOC)
  Gain2/1 -> MATLAB Function/3(Discharge_Limit)

== system Simulation_Fahrmodell_v3/Vehicle Dynamics Model /Drivetrain/Primary and Secondary Axle Powertrain Selector/Primary Axle Powertrain Selector/Hybrid Drive/P3/P3 Motor/Battery and Operating Strategy Limitation (Recuperation)/Begrenzung BAT + Betriebsstrategie EM P2, Reku1 ==
  n_Upmin IN : Inport
  M_Nm : Inport  Port=2
  P_mech_max_kW : Inport  Port=3
  Max1 : MinMax  Function=max  Inputs=2
  "P_kW -> M_Nm" : Subsystem
  n_Upmin OUT : Outport
  M_begr_Nm : Outport  Port=2
  wires:
  M_Nm/1 -> Max1/1
  Max1/1 -> M_begr_Nm/1
  "P_kW -> M_Nm"/1(Out1) -> Max1/2  "M_mech_max_Nm"
  n_Upmin IN/1 -> "P_kW -> M_Nm"/2(In2), n_Upmin OUT/1
  P_mech_max_kW/1 -> "P_kW -> M_Nm"/1(P_kW)  "P_kW"

== system Simulation_Fahrmodell_v3/Vehicle Dynamics Model /Drivetrain/Primary and Secondary Axle Powertrain Selector/Primary Axle Powertrain Selector/Hybrid Drive/P3/P3 Motor/Battery and Operating Strategy Limitation (Recuperation)/Recuperation Limit1 ==
  Torque_Recu_In : Inport
  Constant : Constant  Value=0
  Gain5 : Gain  Gain=100
  Recuperation Limit : Constant  Value=bat.SOC_Recup_Limit
  Relational Operator2 : RelationalOperator  Operator=<  OutDataTypeStr=boolean  RndMeth=Simplest  InputSameDT=off
  Switch2 : Switch  Criteria=u2 > Threshold  SaturateOnIntegerOverflow=off  InputSameDT=off
  Torque_Recu_Out : Outport
  wires:
  Constant/1 -> Switch2/3
  [SOC] -> Relational Operator2/1
  Recuperation Limit/1 -> Gain5/1
  Relational Operator2/1 -> Switch2/2
  Torque_Recu_In/1 -> Switch2/1
  Switch2/1 -> Torque_Recu_Out/1
  Gain5/1 -> Relational Operator2/2

== system Simulation_Fahrmodell_v3/Vehicle Dynamics Model /Drivetrain/Primary and Secondary Axle Powertrain Selector/Secondary Axle Powertrain Selector/Auswahl P4, P4_Dual-Motor/P4 // E2 Single Motor/Battery and Operating Strategy Limitation (Drive)/Begrenzung BAT + Betriebsstrategie EM P4, Fahren1/P_kW -> M_Nm ==
  P_kW : Inport
  In2 : Inport  Port=2
  Constant : Constant
  Constant1 : Constant  Value=2*pi/60/1000
  Divide : Product  Inputs=*//
  Max2 : MinMax  Function=max  Inputs=2
  Out1 : Outport
  wires:
  Divide/1 -> Out1/1
  In2/1 -> Max2/1
  P_kW/1 -> Divide/1
  Constant1/1 -> Divide/2
  Max2/1 -> Divide/3
  Constant/1 -> Max2/2

== system Simulation_Fahrmodell_v3/Vehicle Dynamics Model /Drivetrain/Primary and Secondary Axle Powertrain Selector/Secondary Axle Powertrain Selector/Auswahl P4, P4_Dual-Motor/P4 // E2 Single Motor/Battery and Operating Strategy Limitation (Recuperation)/Begrenzung BAT + Betriebsstrategie EM P4, Reku1/P_kW -> M_Nm ==
  P_kW : Inport
  In2 : Inport  Port=2
  Constant : Constant
  Constant1 : Constant  Value=2*pi/60/1000
  Divide : Product  Inputs=*//
  Max2 : MinMax  Function=max  Inputs=2
  Out1 : Outport
  wires:
  Divide/1 -> Out1/1
  In2/1 -> Max2/1
  P_kW/1 -> Divide/1
  Constant1/1 -> Divide/2
  Max2/1 -> Divide/3
  Constant/1 -> Max2/2

== system Simulation_Fahrmodell_v3/Vehicle Dynamics Model /Drivetrain/Primary and Secondary Axle Powertrain Selector/Secondary Axle Powertrain Selector/Auswahl P4, P4_Dual-Motor/P4 // E3 // E4 Dual Motor/Battery and Operating Strategy Limitation (Drive) 1/Begrenzung BAT + Betriebsstrategie EM P4_DM_L, Fahren1/P_kW -> M_Nm ==
  P_kW : Inport
  In2 : Inport  Port=2
  Constant : Constant
  Constant1 : Constant  Value=2*pi/60/1000
  Divide : Product  Inputs=*//
  Max2 : MinMax  Function=max  Inputs=2
  Out1 : Outport
  wires:
  Divide/1 -> Out1/1
  In2/1 -> Max2/1
  P_kW/1 -> Divide/1
  Constant1/1 -> Divide/2
  Max2/1 -> Divide/3
  Constant/1 -> Max2/2

== system Simulation_Fahrmodell_v3/Vehicle Dynamics Model /Drivetrain/Primary and Secondary Axle Powertrain Selector/Secondary Axle Powertrain Selector/Auswahl P4, P4_Dual-Motor/P4 // E3 // E4 Dual Motor/Battery and Operating Strategy Limitation (Drive) 2/Begrenzung BAT + Betriebsstrategie EM P4_DM_R, Fahren2/P_kW -> M_Nm ==
  P_kW : Inport
  In2 : Inport  Port=2
  Constant : Constant
  Constant1 : Constant  Value=2*pi/60/1000
  Divide : Product  Inputs=*//
  Max2 : MinMax  Function=max  Inputs=2
  Out1 : Outport
  wires:
  Divide/1 -> Out1/1
  In2/1 -> Max2/1
  P_kW/1 -> Divide/1
  Constant1/1 -> Divide/2
  Max2/1 -> Divide/3
  Constant/1 -> Max2/2

== system Simulation_Fahrmodell_v3/Vehicle Dynamics Model /Drivetrain/Primary and Secondary Axle Powertrain Selector/Secondary Axle Powertrain Selector/Auswahl P4, P4_Dual-Motor/P4 // E3 // E4 Dual Motor/Battery and Operating Strategy Limitation (Recuperation) 1/Begrenzung BAT + Betriebsstrategie EM P4_DM_L, Reku1/P_kW -> M_Nm ==
  P_kW : Inport
  In2 : Inport  Port=2
  Constant : Constant
  Constant1 : Constant  Value=2*pi/60/1000
  Divide : Product  Inputs=*//
  Max2 : MinMax  Function=max  Inputs=2
  Out1 : Outport
  wires:
  Divide/1 -> Out1/1
  In2/1 -> Max2/1
  P_kW/1 -> Divide/1
  Constant1/1 -> Divide/2
  Max2/1 -> Divide/3
  Constant/1 -> Max2/2

== system Simulation_Fahrmodell_v3/Vehicle Dynamics Model /Drivetrain/Primary and Secondary Axle Powertrain Selector/Secondary Axle Powertrain Selector/Auswahl P4, P4_Dual-Motor/P4 // E3 // E4 Dual Motor/Battery and Operating Strategy Limitation (Recuperation) 2/Begrenzung BAT + Betriebsstrategie EM P4_DM_R, Reku2/P_kW -> M_Nm ==
  P_kW : Inport
  In2 : Inport  Port=2
  Constant : Constant
  Constant1 : Constant  Value=2*pi/60/1000
  Divide : Product  Inputs=*//
  Max2 : MinMax  Function=max  Inputs=2
  Out1 : Outport
  wires:
  Divide/1 -> Out1/1
  In2/1 -> Max2/1
  P_kW/1 -> Divide/1
  Constant1/1 -> Divide/2
  Max2/1 -> Divide/3
  Constant/1 -> Max2/2

== system Simulation_Fahrmodell_v3/Vehicle Dynamics Model /Drivetrain/Primary and Secondary Axle Powertrain Selector/Primary Axle Powertrain Selector/Electric Drive/Variant Subsystem/EV Dual Motor/Battery and Operating Strategy Limitation (Drive)/Begrenzung BAT + Betriebsstrategie EM P4_DM_L, Fahren2/P_kW -> M_Nm ==
  P_kW : Inport
  In2 : Inport  Port=2
  Constant : Constant
  Constant1 : Constant  Value=2*pi/60/1000
  Divide : Product  Inputs=*//
  Max2 : MinMax  Function=max  Inputs=2
  Out1 : Outport
  wires:
  Divide/1 -> Out1/1
  In2/1 -> Max2/1
  P_kW/1 -> Divide/1
  Constant1/1 -> Divide/2
  Max2/1 -> Divide/3
  Constant/1 -> Max2/2

== system Simulation_Fahrmodell_v3/Vehicle Dynamics Model /Drivetrain/Primary and Secondary Axle Powertrain Selector/Primary Axle Powertrain Selector/Electric Drive/Variant Subsystem/EV Dual Motor/Battery and Operating Strategy Limitation (Drive) /Begrenzung BAT + Betriebsstrategie EM P4_DM_R, Fahren1/P_kW -> M_Nm ==
  P_kW : Inport
  In2 : Inport  Port=2
  Constant : Constant
  Constant1 : Constant  Value=2*pi/60/1000
  Divide : Product  Inputs=*//
  Max2 : MinMax  Function=max  Inputs=2
  Out1 : Outport
  wires:
  Divide/1 -> Out1/1
  In2/1 -> Max2/1
  P_kW/1 -> Divide/1
  Constant1/1 -> Divide/2
  Max2/1 -> Divide/3
  Constant/1 -> Max2/2

== system Simulation_Fahrmodell_v3/Vehicle Dynamics Model /Drivetrain/Primary and Secondary Axle Powertrain Selector/Primary Axle Powertrain Selector/Electric Drive/Variant Subsystem/EV Dual Motor/Battery and Operating Strategy Limitation (Recuperation)/Begrenzung BAT + Betriebsstrategie EM P4_DM_L, Reku2/P_kW -> M_Nm ==
  P_kW : Inport
  In2 : Inport  Port=2
  Constant : Constant
  Constant1 : Constant  Value=2*pi/60/1000
  Divide : Product  Inputs=*//
  Max2 : MinMax  Function=max  Inputs=2
  Out1 : Outport
  wires:
  Divide/1 -> Out1/1
  In2/1 -> Max2/1
  P_kW/1 -> Divide/1
  Constant1/1 -> Divide/2
  Max2/1 -> Divide/3
  Constant/1 -> Max2/2

== system Simulation_Fahrmodell_v3/Vehicle Dynamics Model /Drivetrain/Primary and Secondary Axle Powertrain Selector/Primary Axle Powertrain Selector/Electric Drive/Variant Subsystem/EV Dual Motor/Battery and Operating Strategy Limitation (Recuperation) /Begrenzung BAT + Betriebsstrategie EM P4_DM_R, Reku1/P_kW -> M_Nm ==
  P_kW : Inport
  In2 : Inport  Port=2
  Constant : Constant
  Constant1 : Constant  Value=2*pi/60/1000
  Divide : Product  Inputs=*//
  Max2 : MinMax  Function=max  Inputs=2
  Out1 : Outport
  wires:
  Divide/1 -> Out1/1
  In2/1 -> Max2/1
  P_kW/1 -> Divide/1
  Constant1/1 -> Divide/2
  Max2/1 -> Divide/3
  Constant/1 -> Max2/2

== system Simulation_Fahrmodell_v3/Vehicle Dynamics Model /Drivetrain/Primary and Secondary Axle Powertrain Selector/Primary Axle Powertrain Selector/Electric Drive/Variant Subsystem/EV Single Motor/Battery and Operating Strategy Limitation (Drive)/Begrenzung BAT + Betriebsstrategie EM EV, Fahren2/P_kW -> M_Nm ==
  P_kW : Inport
  In2 : Inport  Port=2
  Constant : Constant
  Constant1 : Constant  Value=2*pi/60/1000
  Divide : Product  Inputs=*//
  Max2 : MinMax  Function=max  Inputs=2
  Out1 : Outport
  wires:
  Divide/1 -> Out1/1
  In2/1 -> Max2/1
  P_kW/1 -> Divide/1
  Constant1/1 -> Divide/2
  Max2/1 -> Divide/3
  Constant/1 -> Max2/2

== system Simulation_Fahrmodell_v3/Vehicle Dynamics Model /Drivetrain/Primary and Secondary Axle Powertrain Selector/Primary Axle Powertrain Selector/Electric Drive/Variant Subsystem/EV Single Motor/Battery and Operating Strategy Limitation (Recuperation)/Begrenzung BAT + Betriebsstrategie EM EV, Reku2/P_kW -> M_Nm ==
  P_kW : Inport
  In2 : Inport  Port=2
  Constant : Constant
  Constant1 : Constant  Value=2*pi/60/1000
  Divide : Product  Inputs=*//
  Max2 : MinMax  Function=max  Inputs=2
  Out1 : Outport
  wires:
  Divide/1 -> Out1/1
  In2/1 -> Max2/1
  P_kW/1 -> Divide/1
  Constant1/1 -> Divide/2
  Max2/1 -> Divide/3
  Constant/1 -> Max2/2

== system Simulation_Fahrmodell_v3/Vehicle Dynamics Model /Drivetrain/Primary and Secondary Axle Powertrain Selector/Primary Axle Powertrain Selector/Hybrid Drive/P0/P0 Motor/Battery and Operating Strategy Limitation (Recuperation)/Begrenzung BAT + Betriebsstrategie EM P2, Reku1/P_kW -> M_Nm ==
  P_kW : Inport
  In2 : Inport  Port=2
  Constant : Constant
  Constant1 : Constant  Value=2*pi/60/1000
  Divide : Product  Inputs=*//
  Max2 : MinMax  Function=max  Inputs=2
  Out1 : Outport
  wires:
  Divide/1 -> Out1/1
  In2/1 -> Max2/1
  P_kW/1 -> Divide/1
  Constant1/1 -> Divide/2
  Max2/1 -> Divide/3
  Constant/1 -> Max2/2

== system Simulation_Fahrmodell_v3/Vehicle Dynamics Model /Drivetrain/Primary and Secondary Axle Powertrain Selector/Primary Axle Powertrain Selector/Hybrid Drive/P0/P0 Motor/SubsysteBattery and Operating Strategy Limitation (Drive)m/Begrenzung BAT + Betriebsstrategie EM P2, Fahren1/P_kW -> M_Nm ==
  P_kW : Inport
  In2 : Inport  Port=2
  Constant : Constant
  Constant1 : Constant  Value=2*pi/60/1000
  Divide : Product  Inputs=*//
  Max2 : MinMax  Function=max  Inputs=2
  Out1 : Outport
  wires:
  Divide/1 -> Out1/1
  In2/1 -> Max2/1
  P_kW/1 -> Divide/1
  Constant1/1 -> Divide/2
  Max2/1 -> Divide/3
  Constant/1 -> Max2/2

== system Simulation_Fahrmodell_v3/Vehicle Dynamics Model /Drivetrain/Primary and Secondary Axle Powertrain Selector/Primary Axle Powertrain Selector/Hybrid Drive/P2/P2 Motor/Battery and Operating Strategy Limitation (Drive)/Begrenzung BAT + Betriebsstrategie EM P2, Fahren1/P_kW -> M_Nm ==
  P_kW : Inport
  In2 : Inport  Port=2
  Constant : Constant
  Constant1 : Constant  Value=2*pi/60/1000
  Divide : Product  Inputs=*//
  Max2 : MinMax  Function=max  Inputs=2
  Out1 : Outport
  wires:
  Divide/1 -> Out1/1
  In2/1 -> Max2/1
  P_kW/1 -> Divide/1
  Constant1/1 -> Divide/2
  Max2/1 -> Divide/3
  Constant/1 -> Max2/2

== system Simulation_Fahrmodell_v3/Vehicle Dynamics Model /Drivetrain/Primary and Secondary Axle Powertrain Selector/Primary Axle Powertrain Selector/Hybrid Drive/P2/P2 Motor/Battery and Operating Strategy Limitation (Recuperation)/Begrenzung BAT + Betriebsstrategie EM P2, Reku1/P_kW -> M_Nm ==
  P_kW : Inport
  In2 : Inport  Port=2
  Constant : Constant
  Constant1 : Constant  Value=2*pi/60/1000
  Divide : Product  Inputs=*//
  Max2 : MinMax  Function=max  Inputs=2
  Out1 : Outport
  wires:
  Divide/1 -> Out1/1
  In2/1 -> Max2/1
  P_kW/1 -> Divide/1
  Constant1/1 -> Divide/2
  Max2/1 -> Divide/3
  Constant/1 -> Max2/2

== system Simulation_Fahrmodell_v3/Vehicle Dynamics Model /Drivetrain/Primary and Secondary Axle Powertrain Selector/Primary Axle Powertrain Selector/Hybrid Drive/P3/P3 Motor/Battery and Operating Strategy Limitation (Drive)/Begrenzung BAT + Betriebsstrategie EM P2, Fahren1/P_kW -> M_Nm ==
  P_kW : Inport
  In2 : Inport  Port=2
  Constant : Constant
  Constant1 : Constant  Value=2*pi/60/1000
  Divide : Product  Inputs=*//
  Max2 : MinMax  Function=max  Inputs=2
  Out1 : Outport
  wires:
  Divide/1 -> Out1/1
  In2/1 -> Max2/1
  P_kW/1 -> Divide/1
  Constant1/1 -> Divide/2
  Max2/1 -> Divide/3
  Constant/1 -> Max2/2

== system Simulation_Fahrmodell_v3/Vehicle Dynamics Model /Drivetrain/Primary and Secondary Axle Powertrain Selector/Primary Axle Powertrain Selector/Hybrid Drive/P3/P3 Motor/Battery and Operating Strategy Limitation (Recuperation)/Begrenzung BAT + Betriebsstrategie EM P2, Reku1/P_kW -> M_Nm ==
  P_kW : Inport
  In2 : Inport  Port=2
  Constant : Constant
  Constant1 : Constant  Value=2*pi/60/1000
  Divide : Product  Inputs=*//
  Max2 : MinMax  Function=max  Inputs=2
  Out1 : Outport
  wires:
  Divide/1 -> Out1/1
  In2/1 -> Max2/1
  P_kW/1 -> Divide/1
  Constant1/1 -> Divide/2
  Max2/1 -> Divide/3
  Constant/1 -> Max2/2
